simulink model "simpleMassSipringDamperModel_matlabFunction"  (R2020b)
settings: Solver=FixedStepAuto  StartTime=0.0  StopTime=10.0  FixedStep=1e-3  RelTol=1e-3
settings Model: Creator=kuzub  LastModifiedBy=kuzub

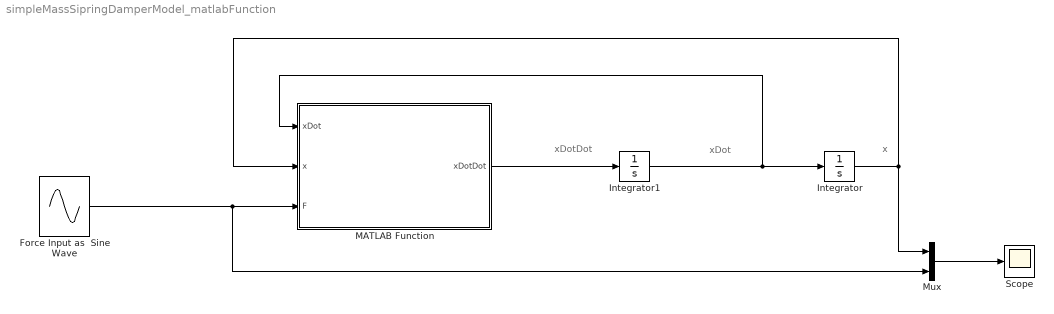
== system simpleMassSipringDamperModel_matlabFunction ==
  note: x
  note: xDot
  note: xDotDot
  Force Input as  Sine Wave : Sin  Amplitude=5  Bias=5  Frequency=2*pi*1  SampleTime=0
  Integrator : Integrator
  Integrator1 : Integrator
  MATLAB Function : MATLAB Function  TreatAsAtomicUnit=on
  Mux : Mux  Inputs=2
  Scope : Scope
  wires:
  MATLAB Function/1(xDotDot) -> Integrator1/1
  Integrator1/1 -> MATLAB Function/1(xDot), Integrator/1
  Integrator/1 -> Mux/1, MATLAB Function/2(x)
  Force Input as  Sine Wave/1 -> Mux/2, MATLAB Function/3(F)
  Mux/1 -> Scope/1

== matlab function simpleMassSipringDamperModel_matlabFunction/MATLAB Function ==
  data: xDot input; xDotDot output; x input; F input
function xDotDot = fcn(xDot, x, F)
%   Constant Variables
    m = 2;  %kg
    c = 2;  %N/ms
    k = 2;  %N/m

    xDotDot_internal = 1/m*(F - k*x - c*xDot);
    
    if xDotDot_internal > 1 
        xDotDot_internal = 0;
    end
    
    xDotDot = xDotDot_internal;
end
